simulink model "dlbsTestHarnessSlice4"  (R2025b)
settings: Solver=VariableStepAuto  StartTime=0.0  StopTime=10.0  RelTol=1e-3
undefined symbols (not defined in the file or in its folder): dY1, dY2, dY3, dY4, X
libraries: dlbsBlockInsertGradientGF x4, dlbsBlockExtractGradientGF x1, dlbsBlockSlice x1
settings Model: Creator=lt6037  LastModifiedBy=lt6037

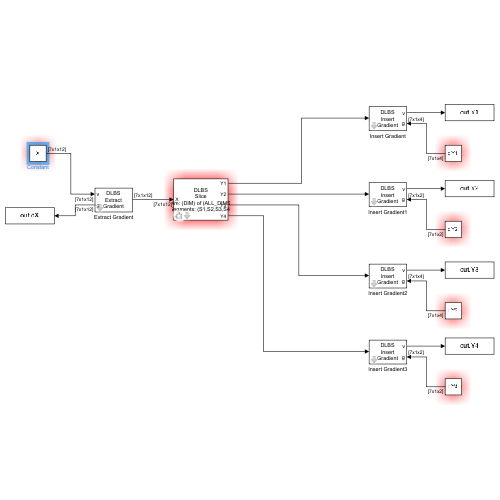
[thumbnail: Simulink's stored preview of the top-level diagram]
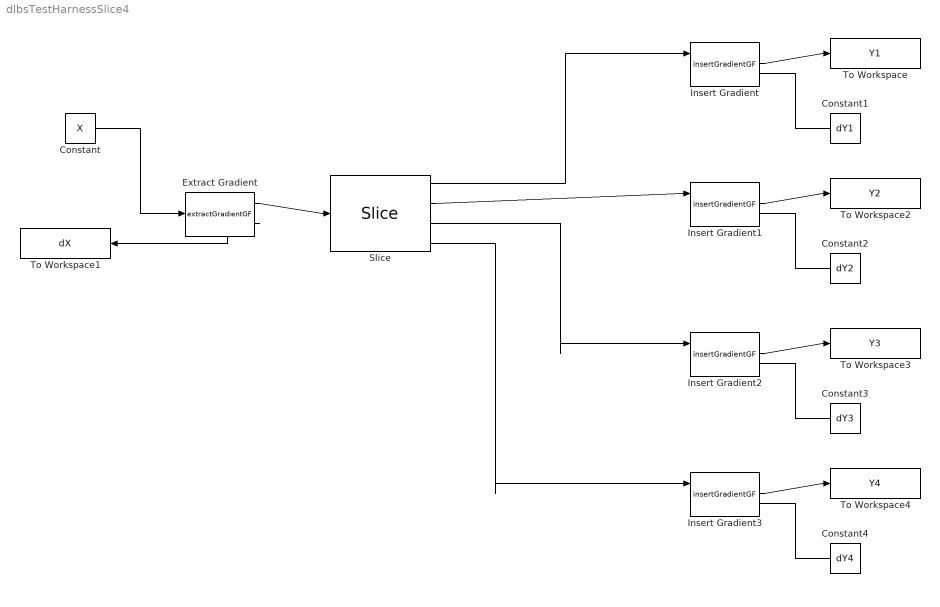
== system dlbsTestHarnessSlice4 ==
  Constant : Constant  Value=X  VectorParams1D=off
  Constant1 : Constant  Value=dY1  VectorParams1D=off
  Constant2 : Constant  Value=dY2  VectorParams1D=off
  Constant3 : Constant  Value=dY3  VectorParams1D=off
  Constant4 : Constant  Value=dY4  VectorParams1D=off
  Extract Gradient : dlbsBlockExtractGradientGF/extractGradientGF
  Insert Gradient{,1..3} (4 alike) : dlbsBlockInsertGradientGF/insertGradientGF
  Slice : dlbsBlockSlice/Slice  n_out=4  all_dims=ALL_DIMS  dim=DIM  s1=S1  s2=S2  s3=S3  s4=S4
  To Workspace : ToWorkspace  VariableName=Y1  SaveFormat=Timeseries  SampleTime=-1
      settings: MaxDataPoints=1
  To Workspace1 : ToWorkspace  VariableName=dX  SaveFormat=Timeseries  SampleTime=-1
      settings: MaxDataPoints=1
  To Workspace2 : ToWorkspace  VariableName=Y2  SaveFormat=Timeseries  SampleTime=-1
      settings: MaxDataPoints=1
  To Workspace3 : ToWorkspace  VariableName=Y3  SaveFormat=Timeseries  SampleTime=-1
      settings: MaxDataPoints=1
  To Workspace4 : ToWorkspace  VariableName=Y4  SaveFormat=Timeseries  SampleTime=-1
      settings: MaxDataPoints=1
  wires:
  Extract Gradient/2 -> To Workspace1/1
  Constant1/1 -> Insert Gradient/2
  Insert Gradient/1 -> To Workspace/1
  Slice/1 -> Insert Gradient/1
  Constant/1 -> Extract Gradient/1
  Extract Gradient/1 -> Slice/1
  Insert Gradient1/1 -> To Workspace2/1
  Constant2/1 -> Insert Gradient1/2
  Constant4/1 -> Insert Gradient3/2
  Insert Gradient3/1 -> To Workspace4/1
  Insert Gradient2/1 -> To Workspace3/1
  Constant3/1 -> Insert Gradient2/2
  Slice/2 -> Insert Gradient1/1
  Slice/3 -> Insert Gradient2/1
  Slice/4 -> Insert Gradient3/1
